simulink model "exemple"  (R2016b)
settings: Solver=VariableStepAuto  StartTime=0.0  StopTime=5  RelTol=1e-3
settings Model: Creator=live  LastModifiedBy=live

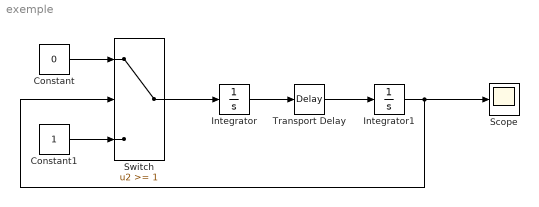
== system exemple ==
  Constant : Constant  Value=0
  Constant1 : Constant
  Integrator : Integrator
  Integrator1 : Integrator
  Scope : Scope
  Switch : Switch  Threshold=1
  Transport Delay : TransportDelay
  wires:
  Constant1/1 -> Switch/3
  Constant/1 -> Switch/1
  Transport Delay/1 -> Integrator1/1
  Integrator/1 -> Transport Delay/1
  Switch/1 -> Integrator/1
  Integrator1/1 -> Scope/1, Switch/2
